simulink model "Punto5"  (R2025b)
settings: Solver=VariableStepAuto  StartTime=0.0  StopTime=0.1  MaxStep=1e-6  RelTol=1e-3
values from neighbouring files (symbols this model uses):
  C = [0 1]    [PROGETTO_CAT_TRACCIA_B_2.m]
  Tout_e = 30.5036    [PROGETTO_CAT_TRACCIA_B_2.m]
  TR_e = 175    [PROGETTO_CAT_TRACCIA_B_2.m]
  u_e = - aR * (Tout_e - TR_e) * KTR_e    (= 771.249535)    [PROGETTO_CAT_TRACCIA_B_2.m]
libraries: cstblocks x1
settings Model: Creator=alex  LastModifiedBy=alex

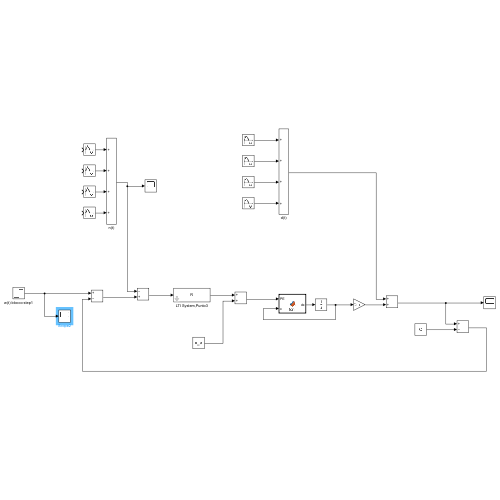
[thumbnail: Simulink's stored preview of the top-level diagram]
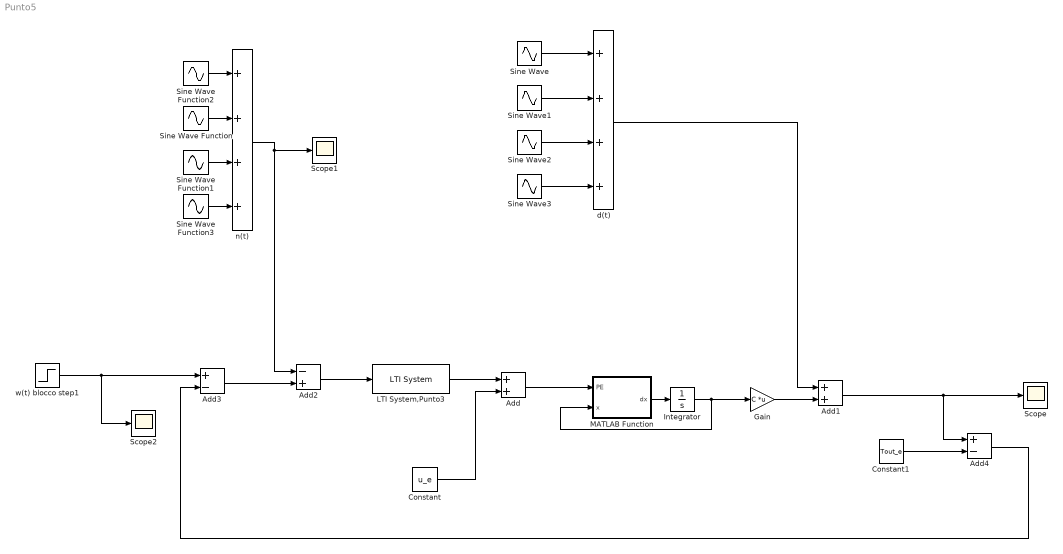
== system Punto5 ==
  Add : Sum
  Add1 : Sum
  Add2 : Sum  Inputs=-+
  Add3 : Sum  Inputs=+-
  Add4 : Sum  Inputs=+-
  Constant : Constant  Value=u_e
  Constant1 : Constant  Value=Tout_e
  Gain : Gain  Gain=C  Multiplication=Matrix(K*u)
  Integrator : Integrator  InitialCondition=[TR_e;Tout_e]
  LTI System,Punto3 : cstblocks/LTI System  sys=R  IC=[]  PadeOrder=0
  MATLAB Function : MATLAB Function  TreatAsAtomicUnit=on
  Scope : Scope
  Scope1 : Scope
      settings: ActiveDisplayYMinimum=-1.1070117590508757  ActiveDisplayYMaximum=1.0601688758437016
  Scope2 : Scope
      settings: ActiveDisplayYMinimum=-1.1070117590508757  ActiveDisplayYMaximum=1.0601688758437016  DataLoggingVariableName=ScopeData2
  Sine Wave : Sin  Amplitude=1.5  Frequency=0.08  SampleTime=0
  Sine Wave Function : Sin  TimeSource=Use external signal  Amplitude=3  Frequency=10e4  SampleTime=0
  Sine Wave Function1 : Sin  TimeSource=Use external signal  Amplitude=3  Frequency=15e4  SampleTime=0
  Sine Wave Function2 : Sin  TimeSource=Use external signal  Amplitude=0  Frequency=5e4  SampleTime=0
  Sine Wave Function3 : Sin  TimeSource=Use external signal  Amplitude=3  Frequency=20e4  SampleTime=0
  Sine Wave1 : Sin  Amplitude=1.5  Frequency=0.16  SampleTime=0
  Sine Wave2 : Sin  Amplitude=1.5  Frequency=0.24  SampleTime=0
  Sine Wave3 : Sin  Amplitude=1.5  Frequency=0.32  SampleTime=0
  d(t) : Sum  Inputs=++++
  n(t) : Sum  Inputs=++++
  w(t) blocco step1 : Step  Time=0  After=4  SampleTime=0
  wires:
  Sine Wave3/1 -> d(t)/4
  w(t) blocco step1/1 -> Scope2/1, Add3/1
  Sine Wave2/1 -> d(t)/3
  Sine Wave1/1 -> d(t)/2
  Sine Wave/1 -> d(t)/1
  Sine Wave Function/1 -> n(t)/2
  Sine Wave Function3/1 -> n(t)/4
  Sine Wave Function1/1 -> n(t)/3
  Sine Wave Function2/1 -> n(t)/1
  MATLAB Function/1(dx) -> Integrator/1
  LTI System,Punto3/1 -> Add/1
  Constant/1 -> Add/2
  Add/1 -> MATLAB Function/1(PE)
  Integrator/1 -> Gain/1, MATLAB Function/2(x)
  d(t)/1 -> Add1/1
  Add2/1 -> LTI System,Punto3/1
  Add3/1 -> Add2/2
  n(t)/1 -> Scope1/1, Add2/1
  Constant1/1 -> Add4/2
  Gain/1 -> Add1/2
  Add1/1 -> Scope/1, Add4/1
  Add4/1 -> Add3/2

== matlab function Punto5/MATLAB Function ==
  data: PE input; dx output; x input
function dx = fcn(PE, x)
    % Parametri fisici [cite: 432]
    hR = 50; AR = 0.07; cR = 840.8; mR = 2.542;
    cA = 1010; mA = 0.1041; m_dotA = 0.2; Tin = 28; kappa = 3e-3;

    % Estrazione degli stati dal vettore x
    % x(1) è TR, x(2) è Tout [cite: 201]
    TR = x(1); 
    Tout = x(2);

    % Equazioni differenziali [cite: 370]
    dTR = ( hR*AR*(Tout - TR) + PE / (1 + kappa*TR) ) / (mR * cR);
    dTout = ( m_dotA*cA*(Tin - Tout) + hR*AR*(TR - Tout) ) / (mA * cA);

    % Output: un unico vettore colonna con le due derivate
    dx = [dTR; dTout];
end
